simulink model "Drone"  (R2020b)
settings: Solver=VariableStepAuto  StartTime=0.0  StopTime=simTime  FixedStep=0.01  RelTol=1e-3
values from neighbouring files (symbols this model uses):
  g = 9.8    [Initialize.m]
  m = drone_params('Mass')    [Initialize.m]
  RPY_init = [0;0;0]    [Initialize.m]
  w_init = [0;0;0]    [Initialize.m]
  XYZ_dot_init = [0;0;0]    [Initialize.m]
  XYZ_init = [0;0;-5]    [Initialize.m]
undefined symbols (not defined in the file or in its folder): commandSig, drone1_gains, drone1_params, stepSize
libraries: pid_lib x6
settings Model: Creator=thang  LastModifiedBy=thang

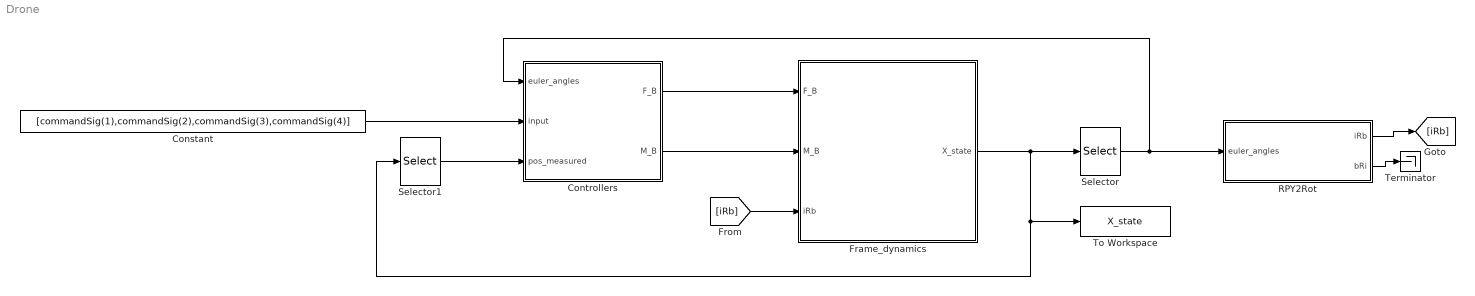
== system Drone ==
  Constant : Constant  Value=[commandSig(1),commandSig(2),commandSig(3),commandSig(4)]
  Controllers : Subsystem
  Frame_dynamics : Subsystem
  RPY2Rot : MATLAB Function  TreatAsAtomicUnit=on
  Selector : Selector  InputPortWidth=12  IndexOptions=Index vector (dialog)  Indices=[7:9]  OutputSizes=1
  Selector1 : Selector  InputPortWidth=12  IndexOptions=Index vector (dialog)  Indices=[1:3]  OutputSizes=1
  Terminator : Terminator
  To Workspace : ToWorkspace  VariableName=X_state  SampleTime=-1
  wires:
  RPY2Rot/1(iRb) -> [iRb]
  [iRb] -> Frame_dynamics/3(iRb)
  Frame_dynamics/1(X_state) -> Selector/1, To Workspace/1, Selector1/1
  Selector/1 -> Controllers/1(euler_angles), RPY2Rot/1(euler_angles)
  RPY2Rot/2(bRi) -> Terminator/1
  Controllers/1(F_B) -> Frame_dynamics/1(F_B)
  Controllers/2(M_B) -> Frame_dynamics/2(M_B)
  Selector1/1 -> Controllers/3(pos_measured)
  Constant/1 -> Controllers/2(input)

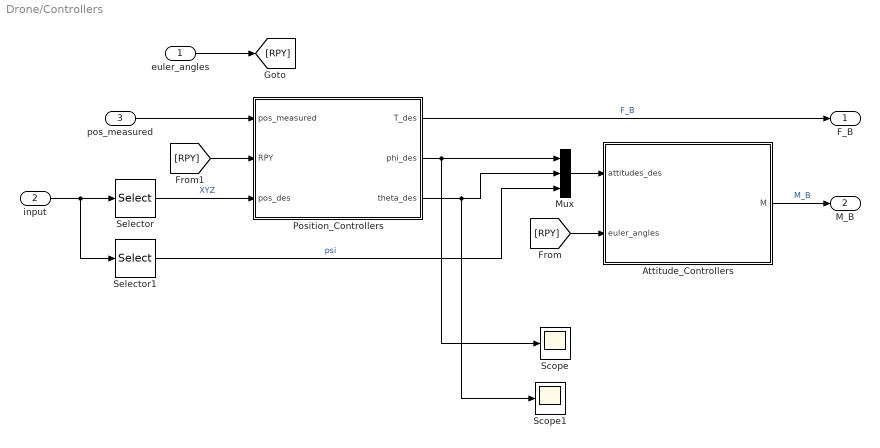
== system Drone/Controllers ==
  euler_angles : Inport
  input : Inport  Port=2
  pos_measured : Inport  Port=3
  Attitude_Controllers : Subsystem
  Mux : Mux  Inputs=3
  Position_Controllers : Subsystem
  Scope : Scope
  Scope1 : Scope
  Selector : Selector  InputPortWidth=4  IndexOptions=Index vector (dialog)  Indices=[1:3]  OutputSizes=1
  Selector1 : Selector  InputPortWidth=4  IndexOptions=Index vector (dialog)  Indices=[4]  OutputSizes=1
  F_B : Outport
  M_B : Outport  Port=2
  wires:
  pos_measured/1 -> Position_Controllers/1(pos_measured)
  Attitude_Controllers/1(M) -> M_B/1  "M_B"
  Position_Controllers/1(T_des) -> F_B/1  "F_B"
  [RPY] -> Attitude_Controllers/2(euler_angles)
  euler_angles/1 -> [RPY]
  [RPY] -> Position_Controllers/2(RPY)
  Mux/1 -> Attitude_Controllers/1(attitudes_des)
  Position_Controllers/2(phi_des) -> Scope/1, Mux/1
  Position_Controllers/3(theta_des) -> Scope1/1, Mux/2
  Selector/1 -> Position_Controllers/3(pos_des)  "XYZ"
  input/1 -> Selector1/1, Selector/1
  Selector1/1 -> Mux/3  "psi"

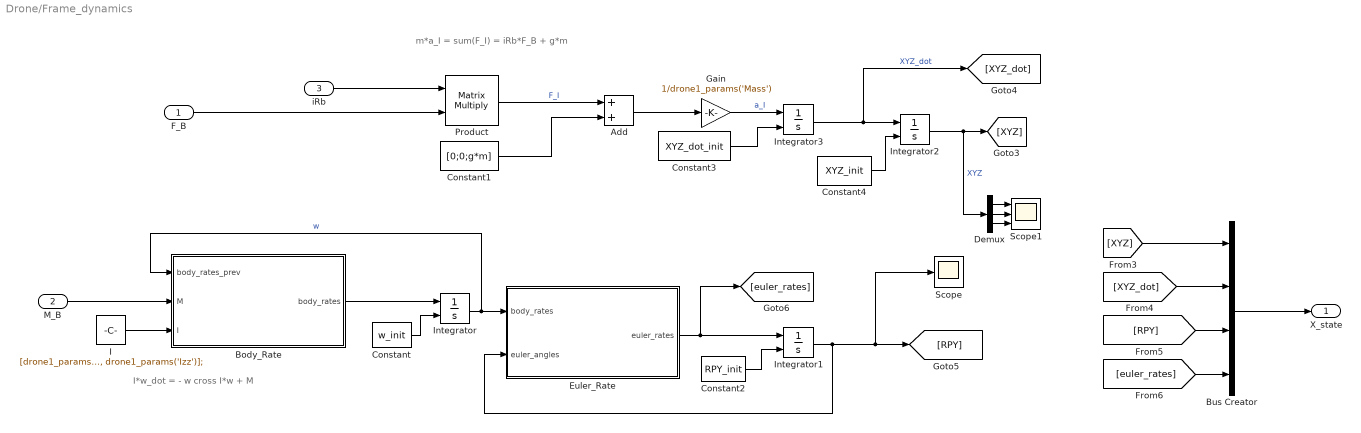
== system Drone/Frame_dynamics ==
  note: I*w_dot = - w cross I*w + M
  note: m*a_I = sum(F_I) = iRb*F_B + g*m
  F_B : Inport
  M_B : Inport  Port=2
  iRb : Inport  Port=3
  Add : Sum
  Body_Rate : MATLAB Function  TreatAsAtomicUnit=on
  Bus Creator : BusCreator  Inputs=4
  Constant : Constant  Value=w_init
  Constant1 : Constant  Value=[0;0;g*m]
  Constant2 : Constant  Value=RPY_init
  Constant3 : Constant  Value=XYZ_dot_init
  Constant4 : Constant  Value=XYZ_init
  Demux : Demux  Outputs=3
  Euler_Rate : MATLAB Function  TreatAsAtomicUnit=on
  Gain : Gain  Gain=1/drone1_params('Mass')
  I : Constant  Value=[drone1_params('Ixx'), 0, 0; 0, drone1_params('Iyy'), 0; 0, 0, drone1_params('Izz')];
  Integrator{,1..3} (4 alike) : Integrator  InitialConditionSource=external
  Product : Product  Multiplication=Matrix(*)
  Scope : Scope
  Scope1 : Scope  NumInputPorts=3
  X_state : Outport
  wires:
  iRb/1 -> Product/1
  F_B/1 -> Product/2
  Product/1 -> Add/1  "F_I"
  Constant1/1 -> Add/2
  Add/1 -> Gain/1
  Gain/1 -> Integrator3/1  "a_I"
  Integrator3/1 -> [XYZ_dot], Integrator2/1  "XYZ_dot"
  Integrator2/1 -> Demux/1, [XYZ]  "XYZ"
  Euler_Rate/1(euler_rates) -> [euler_rates], Integrator1/1
  [XYZ] -> Bus Creator/1
  [XYZ_dot] -> Bus Creator/2
  [RPY] -> Bus Creator/3
  [euler_rates] -> Bus Creator/4
  Bus Creator/1 -> X_state/1
  Integrator1/1 -> Scope/1, [RPY], Euler_Rate/2(euler_angles)
  Integrator/1 -> Euler_Rate/1(body_rates), Body_Rate/1(body_rates_prev)  "w"
  Body_Rate/1(body_rates) -> Integrator/1
  M_B/1 -> Body_Rate/2(M)
  I/1 -> Body_Rate/3(I)
  Constant/1 -> Integrator/2
  Constant2/1 -> Integrator1/2
  Constant3/1 -> Integrator3/2
  Constant4/1 -> Integrator2/2
  Demux/1 -> Scope1/1
  Demux/2 -> Scope1/2
  Demux/3 -> Scope1/3

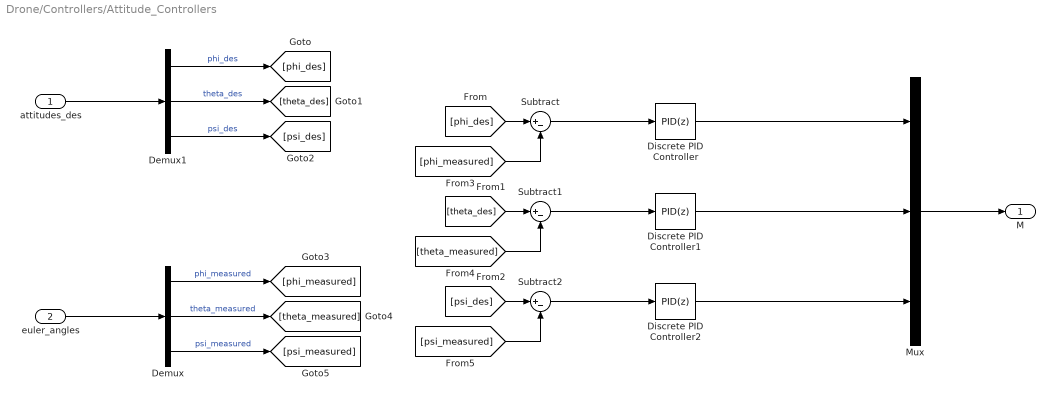
== system Drone/Controllers/Attitude_Controllers ==
  attitudes_des : Inport
  euler_angles : Inport  Port=2
  Demux : Demux  Outputs=3
  Demux1 : Demux  Outputs=3
  Discrete PID Controller : pid_lib/PID Controller  Controller=PID  Form=Parallel  TimeDomain=Discrete-time  UseExternalTs=off  SampleTime=stepSize  IntegratorMethod=Forward Euler  FilterMethod=Forward Euler  ControllerParametersSource=internal  P=drone1_gains('P_phi')  I=drone1_gains('I_phi')  D=drone1_gains('D_phi')  UseFilter=on  N=100  TunerSelectOption=Transfer Function Based (PID Tuner App)  InitialConditionSource=internal  InitialConditionForIntegrator=0  InitialConditionForFilter=0  DifferentiatorICPrevScaledInput=0  ExternalReset=none  TrackingMode=off  Kt=1  LimitOutput=off  SatLimitsSource=internal  UpperSaturationLimit=inf  LowerSaturationLimit=-inf  LinearizeAsGain=off  AntiWindupMode=none  Kb=1  POutMin=[]  POutMax=[]  IOutMin=[]  IOutMax=[]  DOutMin=[]  DOutMax=[]  NOutMin=[]  NOutMax=[]  SumOutMin=[]  SumOutMax=[]  SaturationOutMin=[]  SaturationOutMax=[]  PParamMin=[]  PParamMax=[]  IParamMin=[]  IParamMax=[]  DParamMin=[]  DParamMax=[]  NParamMin=[]  NParamMax=[]  KbParamMin=[]  KbParamMax=[]  KtParamMin=[]  KtParamMax=[]  KbOutMin=[]  KbOutMax=[]  KtOutMin=[]  KtOutMax=[]  IntegratorOutMin=[]  IntegratorOutMax=[]  FilterOutMin=[]  FilterOutMax=[]  SumI1OutMin=[]  SumI1OutMax=[]  SumI2OutMin=[]  SumI2OutMax=[]  SumI3OutMin=[]  SumI3OutMax=[]  SumI4OutMin=[]  SumI4OutMax=[]  SumDOutMin=[]  SumDOutMax=[]  DifferentiatorOutMin=[]  DifferentiatorOutMax=[]  FilterDiffOutCoefMin=[]  FilterDiffOutCoefMax=[]  ReciprocalOutMin=[]  ReciprocalOutMax=[]  SumDenOutMin=[]  SumDenOutMax=[]  SumNumOutMin=[]  SumNumOutMax=[]  DivideOutMin=[]  DivideOutMax=[]  UdiffTsProdOutMin=[]  UdiffTsProdOutMax=[]  NTsProdOutMin=[]  NTsProdOutMax=[]  UintegralTsProdOutMin=[]  UintegralTsProdOutMax=[]  UngainTsProdOutMin=[]  UngainTsProdOutMax=[]  IntegratorContinuousStateAttributes=''  IntegratorStateMustResolveToSignalObject=off  IntegratorRTWStateStorageClass=Auto  FilterContinuousStateAttributes=''  FilterStateMustResolveToSignalObject=off  FilterRTWStateStorageClass=Auto  ParallelPVariant=InternalParameters  IdealPVariant=Disabled  IVariant=InternalParameters  DVariant=InternalParameters  IntegratorVariant=Discrete  SatVariant=Disabled  AWVariant=Passthrough  PCopyVariant=Disabled  TRVariant=Disabled  FdbkBlocksVariant=Forward  IdealPFdbkVariant=Disabled  SatFdbkVariant=Disabled  DerivativeFilterVariant=ForwardEulerFilter  NVariant=InternalParameters  NCopyVariant=Disabled  FilterICVariant=InternalICsFilter  IntegratorICVariant=InternalICs  ExternalResetVariant=Disabled  TRSumVariant=Passthrough  SumFdbkVariant=Disabled  SumVariant=Sum_PID  TsampFilterVariant=InternalTs  TsampNgainVariant=Passthrough  TsampIntegralVariant=Passthrough  ExternalSaturationOutDataTypeStr=Inherit: Same as second input
  Discrete PID Controller1 : pid_lib/PID Controller  Controller=PID  Form=Parallel  TimeDomain=Discrete-time  UseExternalTs=off  SampleTime=stepSize  IntegratorMethod=Forward Euler  FilterMethod=Forward Euler  ControllerParametersSource=internal  P=drone1_gains('P_theta')  I=drone1_gains('I_theta')  D=drone1_gains('D_theta')  UseFilter=on  N=100  TunerSelectOption=Transfer Function Based (PID Tuner App)  InitialConditionSource=internal  InitialConditionForIntegrator=0  InitialConditionForFilter=0  DifferentiatorICPrevScaledInput=0  ExternalReset=none  TrackingMode=off  Kt=1  LimitOutput=off  SatLimitsSource=internal  UpperSaturationLimit=inf  LowerSaturationLimit=-inf  LinearizeAsGain=off  AntiWindupMode=none  Kb=1  POutMin=[]  POutMax=[]  IOutMin=[]  IOutMax=[]  DOutMin=[]  DOutMax=[]  NOutMin=[]  NOutMax=[]  SumOutMin=[]  SumOutMax=[]  SaturationOutMin=[]  SaturationOutMax=[]  PParamMin=[]  PParamMax=[]  IParamMin=[]  IParamMax=[]  DParamMin=[]  DParamMax=[]  NParamMin=[]  NParamMax=[]  KbParamMin=[]  KbParamMax=[]  KtParamMin=[]  KtParamMax=[]  KbOutMin=[]  KbOutMax=[]  KtOutMin=[]  KtOutMax=[]  IntegratorOutMin=[]  IntegratorOutMax=[]  FilterOutMin=[]  FilterOutMax=[]  SumI1OutMin=[]  SumI1OutMax=[]  SumI2OutMin=[]  SumI2OutMax=[]  SumI3OutMin=[]  SumI3OutMax=[]  SumI4OutMin=[]  SumI4OutMax=[]  SumDOutMin=[]  SumDOutMax=[]  DifferentiatorOutMin=[]  DifferentiatorOutMax=[]  FilterDiffOutCoefMin=[]  FilterDiffOutCoefMax=[]  ReciprocalOutMin=[]  ReciprocalOutMax=[]  SumDenOutMin=[]  SumDenOutMax=[]  SumNumOutMin=[]  SumNumOutMax=[]  DivideOutMin=[]  DivideOutMax=[]  UdiffTsProdOutMin=[]  UdiffTsProdOutMax=[]  NTsProdOutMin=[]  NTsProdOutMax=[]  UintegralTsProdOutMin=[]  UintegralTsProdOutMax=[]  UngainTsProdOutMin=[]  UngainTsProdOutMax=[]  IntegratorContinuousStateAttributes=''  IntegratorStateMustResolveToSignalObject=off  IntegratorRTWStateStorageClass=Auto  FilterContinuousStateAttributes=''  FilterStateMustResolveToSignalObject=off  FilterRTWStateStorageClass=Auto  ParallelPVariant=InternalParameters  IdealPVariant=Disabled  IVariant=InternalParameters  DVariant=InternalParameters  IntegratorVariant=Discrete  SatVariant=Disabled  AWVariant=Passthrough  PCopyVariant=Disabled  TRVariant=Disabled  FdbkBlocksVariant=Forward  IdealPFdbkVariant=Disabled  SatFdbkVariant=Disabled  DerivativeFilterVariant=ForwardEulerFilter  NVariant=InternalParameters  NCopyVariant=Disabled  FilterICVariant=InternalICsFilter  IntegratorICVariant=InternalICs  ExternalResetVariant=Disabled  TRSumVariant=Passthrough  SumFdbkVariant=Disabled  SumVariant=Sum_PID  TsampFilterVariant=InternalTs  TsampNgainVariant=Passthrough  TsampIntegralVariant=Passthrough  ExternalSaturationOutDataTypeStr=Inherit: Same as second input
  Discrete PID Controller2 : pid_lib/PID Controller  Controller=PID  Form=Parallel  TimeDomain=Discrete-time  UseExternalTs=off  SampleTime=stepSize  IntegratorMethod=Forward Euler  FilterMethod=Forward Euler  ControllerParametersSource=internal  P=drone1_gains('P_psi')  I=drone1_gains('I_psi')  D=drone1_gains('D_psi')  UseFilter=on  N=100  TunerSelectOption=Transfer Function Based (PID Tuner App)  InitialConditionSource=internal  InitialConditionForIntegrator=0  InitialConditionForFilter=0  DifferentiatorICPrevScaledInput=0  ExternalReset=none  TrackingMode=off  Kt=1  LimitOutput=off  SatLimitsSource=internal  UpperSaturationLimit=inf  LowerSaturationLimit=-inf  LinearizeAsGain=off  AntiWindupMode=none  Kb=1  POutMin=[]  POutMax=[]  IOutMin=[]  IOutMax=[]  DOutMin=[]  DOutMax=[]  NOutMin=[]  NOutMax=[]  SumOutMin=[]  SumOutMax=[]  SaturationOutMin=[]  SaturationOutMax=[]  PParamMin=[]  PParamMax=[]  IParamMin=[]  IParamMax=[]  DParamMin=[]  DParamMax=[]  NParamMin=[]  NParamMax=[]  KbParamMin=[]  KbParamMax=[]  KtParamMin=[]  KtParamMax=[]  KbOutMin=[]  KbOutMax=[]  KtOutMin=[]  KtOutMax=[]  IntegratorOutMin=[]  IntegratorOutMax=[]  FilterOutMin=[]  FilterOutMax=[]  SumI1OutMin=[]  SumI1OutMax=[]  SumI2OutMin=[]  SumI2OutMax=[]  SumI3OutMin=[]  SumI3OutMax=[]  SumI4OutMin=[]  SumI4OutMax=[]  SumDOutMin=[]  SumDOutMax=[]  DifferentiatorOutMin=[]  DifferentiatorOutMax=[]  FilterDiffOutCoefMin=[]  FilterDiffOutCoefMax=[]  ReciprocalOutMin=[]  ReciprocalOutMax=[]  SumDenOutMin=[]  SumDenOutMax=[]  SumNumOutMin=[]  SumNumOutMax=[]  DivideOutMin=[]  DivideOutMax=[]  UdiffTsProdOutMin=[]  UdiffTsProdOutMax=[]  NTsProdOutMin=[]  NTsProdOutMax=[]  UintegralTsProdOutMin=[]  UintegralTsProdOutMax=[]  UngainTsProdOutMin=[]  UngainTsProdOutMax=[]  IntegratorContinuousStateAttributes=''  IntegratorStateMustResolveToSignalObject=off  IntegratorRTWStateStorageClass=Auto  FilterContinuousStateAttributes=''  FilterStateMustResolveToSignalObject=off  FilterRTWStateStorageClass=Auto  ParallelPVariant=InternalParameters  IdealPVariant=Disabled  IVariant=InternalParameters  DVariant=InternalParameters  IntegratorVariant=Discrete  SatVariant=Disabled  AWVariant=Passthrough  PCopyVariant=Disabled  TRVariant=Disabled  FdbkBlocksVariant=Forward  IdealPFdbkVariant=Disabled  SatFdbkVariant=Disabled  DerivativeFilterVariant=ForwardEulerFilter  NVariant=InternalParameters  NCopyVariant=Disabled  FilterICVariant=InternalICsFilter  IntegratorICVariant=InternalICs  ExternalResetVariant=Disabled  TRSumVariant=Passthrough  SumFdbkVariant=Disabled  SumVariant=Sum_PID  TsampFilterVariant=InternalTs  TsampNgainVariant=Passthrough  TsampIntegralVariant=Passthrough  ExternalSaturationOutDataTypeStr=Inherit: Same as second input
  Mux : Mux  Inputs=3
  Subtract : Sum  Inputs=|+-
  Subtract1 : Sum  Inputs=|+-
  Subtract2 : Sum  Inputs=|+-
  M : Outport
  wires:
  attitudes_des/1 -> Demux1/1
  euler_angles/1 -> Demux/1
  Demux/1 -> [phi_measured]  "phi_measured"
  Demux/2 -> [theta_measured]  "theta_measured"
  Demux/3 -> [psi_measured]  "psi_measured"
  Demux1/1 -> [phi_des]  "phi_des"
  Demux1/2 -> [theta_des]  "theta_des"
  Demux1/3 -> [psi_des]  "psi_des"
  [phi_des] -> Subtract/1
  Subtract/1 -> Discrete PID Controller/1
  [phi_measured] -> Subtract/2
  Subtract1/1 -> Discrete PID Controller1/1
  Discrete PID Controller1/1 -> Mux/2
  [theta_measured] -> Subtract1/2
  [theta_des] -> Subtract1/1
  Subtract2/1 -> Discrete PID Controller2/1
  Discrete PID Controller2/1 -> Mux/3
  [psi_measured] -> Subtract2/2
  [psi_des] -> Subtract2/1
  Discrete PID Controller/1 -> Mux/1
  Mux/1 -> M/1

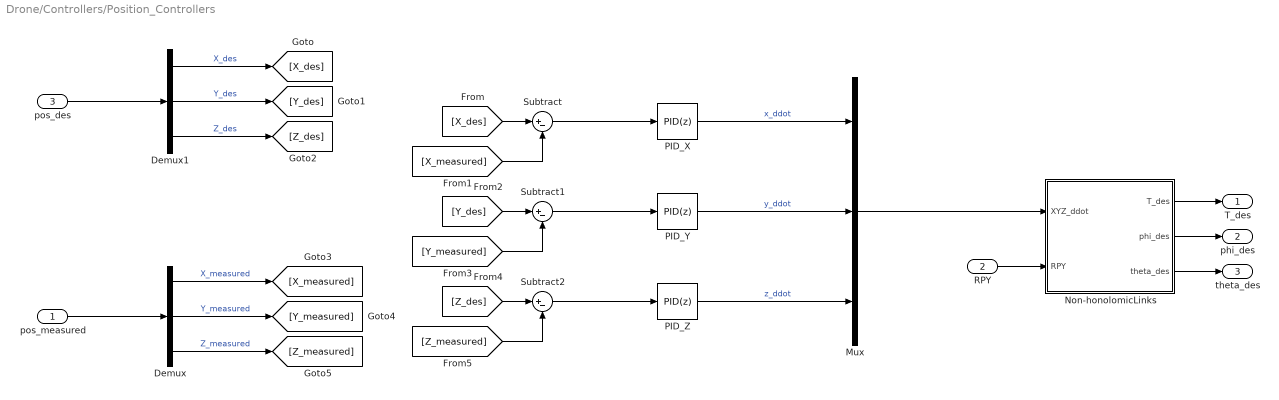
== system Drone/Controllers/Position_Controllers ==
  pos_measured : Inport
  RPY : Inport  Port=2
  pos_des : Inport  Port=3
  Demux : Demux  Outputs=3
  Demux1 : Demux  Outputs=3
  Mux : Mux  Inputs=3
  Non-honolomicLinks : MATLAB Function  TreatAsAtomicUnit=on
  PID_X : pid_lib/PID Controller  Controller=PID  Form=Parallel  TimeDomain=Discrete-time  UseExternalTs=off  SampleTime=stepSize  IntegratorMethod=Forward Euler  FilterMethod=Forward Euler  ControllerParametersSource=internal  P=drone1_gains('P_x')  I=drone1_gains('I_x')  D=drone1_gains('D_x')  UseFilter=on  N=100  TunerSelectOption=Transfer Function Based (PID Tuner App)  InitialConditionSource=internal  InitialConditionForIntegrator=0  InitialConditionForFilter=0  DifferentiatorICPrevScaledInput=0  ExternalReset=none  TrackingMode=off  Kt=1  LimitOutput=off  SatLimitsSource=internal  UpperSaturationLimit=inf  LowerSaturationLimit=-inf  LinearizeAsGain=off  AntiWindupMode=none  Kb=1  POutMin=[]  POutMax=[]  IOutMin=[]  IOutMax=[]  DOutMin=[]  DOutMax=[]  NOutMin=[]  NOutMax=[]  SumOutMin=[]  SumOutMax=[]  SaturationOutMin=[]  SaturationOutMax=[]  PParamMin=[]  PParamMax=[]  IParamMin=[]  IParamMax=[]  DParamMin=[]  DParamMax=[]  NParamMin=[]  NParamMax=[]  KbParamMin=[]  KbParamMax=[]  KtParamMin=[]  KtParamMax=[]  KbOutMin=[]  KbOutMax=[]  KtOutMin=[]  KtOutMax=[]  IntegratorOutMin=[]  IntegratorOutMax=[]  FilterOutMin=[]  FilterOutMax=[]  SumI1OutMin=[]  SumI1OutMax=[]  SumI2OutMin=[]  SumI2OutMax=[]  SumI3OutMin=[]  SumI3OutMax=[]  SumI4OutMin=[]  SumI4OutMax=[]  SumDOutMin=[]  SumDOutMax=[]  DifferentiatorOutMin=[]  DifferentiatorOutMax=[]  FilterDiffOutCoefMin=[]  FilterDiffOutCoefMax=[]  ReciprocalOutMin=[]  ReciprocalOutMax=[]  SumDenOutMin=[]  SumDenOutMax=[]  SumNumOutMin=[]  SumNumOutMax=[]  DivideOutMin=[]  DivideOutMax=[]  UdiffTsProdOutMin=[]  UdiffTsProdOutMax=[]  NTsProdOutMin=[]  NTsProdOutMax=[]  UintegralTsProdOutMin=[]  UintegralTsProdOutMax=[]  UngainTsProdOutMin=[]  UngainTsProdOutMax=[]  IntegratorContinuousStateAttributes=''  IntegratorStateMustResolveToSignalObject=off  IntegratorRTWStateStorageClass=Auto  FilterContinuousStateAttributes=''  FilterStateMustResolveToSignalObject=off  FilterRTWStateStorageClass=Auto  ParallelPVariant=InternalParameters  IdealPVariant=Disabled  IVariant=InternalParameters  DVariant=InternalParameters  IntegratorVariant=Discrete  SatVariant=Disabled  AWVariant=Passthrough  PCopyVariant=Disabled  TRVariant=Disabled  FdbkBlocksVariant=Forward  IdealPFdbkVariant=Disabled  SatFdbkVariant=Disabled  DerivativeFilterVariant=ForwardEulerFilter  NVariant=InternalParameters  NCopyVariant=Disabled  FilterICVariant=InternalICsFilter  IntegratorICVariant=InternalICs  ExternalResetVariant=Disabled  TRSumVariant=Passthrough  SumFdbkVariant=Disabled  SumVariant=Sum_PID  TsampFilterVariant=InternalTs  TsampNgainVariant=Passthrough  TsampIntegralVariant=Passthrough  ExternalSaturationOutDataTypeStr=Inherit: Same as second input
  PID_Y : pid_lib/PID Controller  Controller=PID  Form=Parallel  TimeDomain=Discrete-time  UseExternalTs=off  SampleTime=stepSize  IntegratorMethod=Forward Euler  FilterMethod=Forward Euler  ControllerParametersSource=internal  P=drone1_gains('P_y')  I=drone1_gains('I_y')  D=drone1_gains('D_y')  UseFilter=on  N=100  TunerSelectOption=Transfer Function Based (PID Tuner App)  InitialConditionSource=internal  InitialConditionForIntegrator=0  InitialConditionForFilter=0  DifferentiatorICPrevScaledInput=0  ExternalReset=none  TrackingMode=off  Kt=1  LimitOutput=off  SatLimitsSource=internal  UpperSaturationLimit=inf  LowerSaturationLimit=-inf  LinearizeAsGain=off  AntiWindupMode=none  Kb=1  POutMin=[]  POutMax=[]  IOutMin=[]  IOutMax=[]  DOutMin=[]  DOutMax=[]  NOutMin=[]  NOutMax=[]  SumOutMin=[]  SumOutMax=[]  SaturationOutMin=[]  SaturationOutMax=[]  PParamMin=[]  PParamMax=[]  IParamMin=[]  IParamMax=[]  DParamMin=[]  DParamMax=[]  NParamMin=[]  NParamMax=[]  KbParamMin=[]  KbParamMax=[]  KtParamMin=[]  KtParamMax=[]  KbOutMin=[]  KbOutMax=[]  KtOutMin=[]  KtOutMax=[]  IntegratorOutMin=[]  IntegratorOutMax=[]  FilterOutMin=[]  FilterOutMax=[]  SumI1OutMin=[]  SumI1OutMax=[]  SumI2OutMin=[]  SumI2OutMax=[]  SumI3OutMin=[]  SumI3OutMax=[]  SumI4OutMin=[]  SumI4OutMax=[]  SumDOutMin=[]  SumDOutMax=[]  DifferentiatorOutMin=[]  DifferentiatorOutMax=[]  FilterDiffOutCoefMin=[]  FilterDiffOutCoefMax=[]  ReciprocalOutMin=[]  ReciprocalOutMax=[]  SumDenOutMin=[]  SumDenOutMax=[]  SumNumOutMin=[]  SumNumOutMax=[]  DivideOutMin=[]  DivideOutMax=[]  UdiffTsProdOutMin=[]  UdiffTsProdOutMax=[]  NTsProdOutMin=[]  NTsProdOutMax=[]  UintegralTsProdOutMin=[]  UintegralTsProdOutMax=[]  UngainTsProdOutMin=[]  UngainTsProdOutMax=[]  IntegratorContinuousStateAttributes=''  IntegratorStateMustResolveToSignalObject=off  IntegratorRTWStateStorageClass=Auto  FilterContinuousStateAttributes=''  FilterStateMustResolveToSignalObject=off  FilterRTWStateStorageClass=Auto  ParallelPVariant=InternalParameters  IdealPVariant=Disabled  IVariant=InternalParameters  DVariant=InternalParameters  IntegratorVariant=Discrete  SatVariant=Disabled  AWVariant=Passthrough  PCopyVariant=Disabled  TRVariant=Disabled  FdbkBlocksVariant=Forward  IdealPFdbkVariant=Disabled  SatFdbkVariant=Disabled  DerivativeFilterVariant=ForwardEulerFilter  NVariant=InternalParameters  NCopyVariant=Disabled  FilterICVariant=InternalICsFilter  IntegratorICVariant=InternalICs  ExternalResetVariant=Disabled  TRSumVariant=Passthrough  SumFdbkVariant=Disabled  SumVariant=Sum_PID  TsampFilterVariant=InternalTs  TsampNgainVariant=Passthrough  TsampIntegralVariant=Passthrough  ExternalSaturationOutDataTypeStr=Inherit: Same as second input
  PID_Z : pid_lib/PID Controller  Controller=PID  Form=Parallel  TimeDomain=Discrete-time  UseExternalTs=off  SampleTime=stepSize  IntegratorMethod=Forward Euler  FilterMethod=Forward Euler  ControllerParametersSource=internal  P=drone1_gains('P_z')  I=drone1_gains('I_z')  D=drone1_gains('D_z')  UseFilter=on  N=100  TunerSelectOption=Transfer Function Based (PID Tuner App)  InitialConditionSource=internal  InitialConditionForIntegrator=0  InitialConditionForFilter=0  DifferentiatorICPrevScaledInput=0  ExternalReset=none  TrackingMode=off  Kt=1  LimitOutput=off  SatLimitsSource=internal  UpperSaturationLimit=inf  LowerSaturationLimit=-inf  LinearizeAsGain=off  AntiWindupMode=none  Kb=1  POutMin=[]  POutMax=[]  IOutMin=[]  IOutMax=[]  DOutMin=[]  DOutMax=[]  NOutMin=[]  NOutMax=[]  SumOutMin=[]  SumOutMax=[]  SaturationOutMin=[]  SaturationOutMax=[]  PParamMin=[]  PParamMax=[]  IParamMin=[]  IParamMax=[]  DParamMin=[]  DParamMax=[]  NParamMin=[]  NParamMax=[]  KbParamMin=[]  KbParamMax=[]  KtParamMin=[]  KtParamMax=[]  KbOutMin=[]  KbOutMax=[]  KtOutMin=[]  KtOutMax=[]  IntegratorOutMin=[]  IntegratorOutMax=[]  FilterOutMin=[]  FilterOutMax=[]  SumI1OutMin=[]  SumI1OutMax=[]  SumI2OutMin=[]  SumI2OutMax=[]  SumI3OutMin=[]  SumI3OutMax=[]  SumI4OutMin=[]  SumI4OutMax=[]  SumDOutMin=[]  SumDOutMax=[]  DifferentiatorOutMin=[]  DifferentiatorOutMax=[]  FilterDiffOutCoefMin=[]  FilterDiffOutCoefMax=[]  ReciprocalOutMin=[]  ReciprocalOutMax=[]  SumDenOutMin=[]  SumDenOutMax=[]  SumNumOutMin=[]  SumNumOutMax=[]  DivideOutMin=[]  DivideOutMax=[]  UdiffTsProdOutMin=[]  UdiffTsProdOutMax=[]  NTsProdOutMin=[]  NTsProdOutMax=[]  UintegralTsProdOutMin=[]  UintegralTsProdOutMax=[]  UngainTsProdOutMin=[]  UngainTsProdOutMax=[]  IntegratorContinuousStateAttributes=''  IntegratorStateMustResolveToSignalObject=off  IntegratorRTWStateStorageClass=Auto  FilterContinuousStateAttributes=''  FilterStateMustResolveToSignalObject=off  FilterRTWStateStorageClass=Auto  ParallelPVariant=InternalParameters  IdealPVariant=Disabled  IVariant=InternalParameters  DVariant=InternalParameters  IntegratorVariant=Discrete  SatVariant=Disabled  AWVariant=Passthrough  PCopyVariant=Disabled  TRVariant=Disabled  FdbkBlocksVariant=Forward  IdealPFdbkVariant=Disabled  SatFdbkVariant=Disabled  DerivativeFilterVariant=ForwardEulerFilter  NVariant=InternalParameters  NCopyVariant=Disabled  FilterICVariant=InternalICsFilter  IntegratorICVariant=InternalICs  ExternalResetVariant=Disabled  TRSumVariant=Passthrough  SumFdbkVariant=Disabled  SumVariant=Sum_PID  TsampFilterVariant=InternalTs  TsampNgainVariant=Passthrough  TsampIntegralVariant=Passthrough  ExternalSaturationOutDataTypeStr=Inherit: Same as second input
  Subtract : Sum  Inputs=|+-
  Subtract1 : Sum  Inputs=|+-
  Subtract2 : Sum  Inputs=|+-
  T_des : Outport
  phi_des : Outport  Port=2
  theta_des : Outport  Port=3
  wires:
  PID_X/1 -> Mux/1  "x_ddot"
  [Z_des] -> Subtract2/1
  [Z_measured] -> Subtract2/2
  PID_Z/1 -> Mux/3  "z_ddot"
  Subtract2/1 -> PID_Z/1
  [Y_des] -> Subtract1/1
  [Y_measured] -> Subtract1/2
  PID_Y/1 -> Mux/2  "y_ddot"
  Subtract1/1 -> PID_Y/1
  [X_measured] -> Subtract/2
  Subtract/1 -> PID_X/1
  [X_des] -> Subtract/1
  Demux1/3 -> [Z_des]  "Z_des"
  Demux1/2 -> [Y_des]  "Y_des"
  Demux1/1 -> [X_des]  "X_des"
  Demux/3 -> [Z_measured]  "Z_measured"
  Demux/2 -> [Y_measured]  "Y_measured"
  Demux/1 -> [X_measured]  "X_measured"
  pos_measured/1 -> Demux/1
  pos_des/1 -> Demux1/1
  Non-honolomicLinks/1(T_des) -> T_des/1
  Non-honolomicLinks/2(phi_des) -> phi_des/1
  Non-honolomicLinks/3(theta_des) -> theta_des/1
  RPY/1 -> Non-honolomicLinks/2(RPY)
  Mux/1 -> Non-honolomicLinks/1(XYZ_ddot)

== matlab function Drone/Frame_dynamics/Euler_Rate ==
  data: body_rates input; euler_angles input; euler_rates output size=3
function  euler_rates = fcn(body_rates, euler_angles)
    phi = euler_angles(1);
    theta = euler_angles(2);
    
    euler_rates = [1 sin(phi)*tan(theta) cos(phi)*tan(theta);...
                   0 cos(phi) -sin(phi);...
                   0 sin(phi)/cos(theta) cos(phi)/cos(theta)] * body_rates;

== matlab function Drone/RPY2Rot ==
  data: euler_angles input; iRb output; bRi output
function [iRb, bRi] = fcn(euler_angles)
    phi = euler_angles(1);
    theta = euler_angles(2);
    psi = euler_angles(3);
    
    R_psi =   [ cos(psi)  sin(psi) 0; ...
                -sin(psi) cos(psi) 0; ...
                0         0        1];
    R_theta = [ cos(theta)  0    -sin(theta); ...
                0           1              0; ...
                sin(theta)  0     cos(theta)];
    R_phi =   [ 1          0            0; ...
                0   cos(phi)     sin(phi); ...
                0  -sin(phi)     cos(phi)];
    
    % Yaw, Pitch, Roll sequence
    bRi = R_phi * R_theta * R_psi;
    iRb = bRi';

== matlab function Drone/Frame_dynamics/Body_Rate ==
  data: body_rates_prev input; M input; I input; body_rates output size=3
function  body_rates = fcn(body_rates_prev, M, I)
    body_rates = I \ (M - cross(body_rates_prev, I * body_rates_prev));

== matlab function Drone/Controllers/Position_Controllers/Non-honolomicLinks ==
  data: XYZ_ddot input size=3; T_des output; RPY input; phi_des output; theta_des output

function [T_des, phi_des, theta_des] = fcn(XYZ_ddot, RPY)
    X_ddot = XYZ_ddot(1);
    Y_ddot = XYZ_ddot(2);
    Z_ddot = XYZ_ddot(3);
    m = 1.25;
    g = 9.8;
    psi = RPY(3);

    T_des = [0;0;- m / sqrt(X_ddot^2 + Y_ddot^2 + (Z_ddot + g)^2)];

    phi_des = asin((X_ddot*sin(psi) - Y_ddot*cos(psi)) / sqrt(X_ddot^2 + Y_ddot^2 + (Z_ddot + g)^2));

    theta_des = atan((X_ddot*cos(psi) + Y_ddot*sin(psi))/ (Z_ddot + g));
